simulink model "AttitudeKalman"  (Simulink 6.6)
settings: Solver=ode4  StartTime=0.0  StopTime=500  FixedStep=SampleT  RelTol=1e-3
InitFcn:
  | clc
  | Taxi_Var
  | failures
  | insInit
values from neighbouring files (symbols this model uses):
  A1 = 0    [Taxi_Var.m]    (also in Taxi_Var_new.m = 0.007)
  Apolar = 0.0899    [Taxi_Var.m]    (also in Taxi_Var_new.m = 0.057)
  APtsamp = 0.005    [failures.m]    (also in piccolo_init.m = 0.05)
  b0 = [0.01 0.01 0.01]    [insInit.m]
  CD0 = 0.0219    [Taxi_Var.m]    (also in Taxi_Var_new.m = 0.022)
  chord = S/span    (= 0.384036716878)    [Taxi_Var.m]    (also in Taxi_Var_new.m = 0.351341681574)
  CL0 = 0.1857    [Taxi_Var.m]    (also in Taxi_Var_new.m = 0.38)
  CLa = 4.6206    [Taxi_Var.m]    (also in Taxi_Var_new.m = 18.5)
  CLa_dot = 1.93    [Taxi_Var.m]    (also in Taxi_Var_new.m = 2.64)
  Clb = -0.0043    [Taxi_Var.m]    (also in Taxi_Var_new.m = -0.06)
  ClDa = 0.1695    [Taxi_Var.m]    (also in Taxi_Var_new.m)
  CLDe = 0.4032    [Taxi_Var.m]    (also in Taxi_Var_new.m = 0.24)
  CLDf = 0.047    [Taxi_Var.m]    (also in Taxi_Var_new.m = 0.4)
  ClDr = 0.0003    [Taxi_Var.m]    (also in Taxi_Var_new.m = 0.055)
  Clp = -0.4425    [Taxi_Var.m]    (also in Taxi_Var_new.m = -0.88)
  CLq = 8.7465    [Taxi_Var.m]    (also in Taxi_Var_new.m = 7.4)
  Clr = 0.0675    [Taxi_Var.m]    (also in Taxi_Var_new.m = 0.04)
  Cm0 = -0.0902    [Taxi_Var.m]    (also in Taxi_Var_new.m = 0.56)
  Cm0_factor = 0.9    [failures.m]
  Cm0_fail = 0    [failures.m]
  Cma = -1.3995    [Taxi_Var.m]    (also in Taxi_Var_new.m = -1.58)
  CmDe = -0.9493    [Taxi_Var.m]    (also in Taxi_Var_new.m = -41)
  CmDf = -.021    (= -0.021)    [Taxi_Var.m]    (also in Taxi_Var_new.m)
  Cnb = 0.0281    [Taxi_Var.m]    (also in Taxi_Var_new.m = 0.73)
  CnDa = -0.0031    [Taxi_Var.m]    (also in Taxi_Var_new.m = -0.032)
  CnDr = -0.0882    [Taxi_Var.m]    (also in Taxi_Var_new.m = 0.19)
  Cnp = -0.0695    [Taxi_Var.m]    (also in Taxi_Var_new.m = -0.1)
  Cnr = -0.1045    [Taxi_Var.m]    (also in Taxi_Var_new.m = -0.23)
  CYb = -0.1999    [Taxi_Var.m]    (also in Taxi_Var_new.m = -0.98)
  CYDr = 0.0192    [Taxi_Var.m]    (also in Taxi_Var_new.m = 0.066)
  da_failamp = 5    [failures.m]
  da_failbias = -da_failamp/2    (= -2.5)    [failures.m]
  da_failper = 90    [failures.m]
  daL_fail = 0    [failures.m]
  daR_fail = 0    [failures.m]
  dr_fail = 0    [failures.m]
  dr_failamp = 2    [failures.m]
  dr_failbias = -dr_failamp/2    (= -1)    [failures.m]
  dr_failper = 70    [failures.m]
  Euler_0 = [0; 0; 45]'*pi/180    [Taxi_Var.m]    (also in Taxi_Var_new.m = [0 0 45]'*pi/180)
  Gw = zeros(6,6)    [insInit.m]
  H = [eye(3,3) zeros(3,3)]    [insInit.m]
  ISA_g = 9.815    [Taxi_Var.m]    (also in Taxi_Var_new.m)
  Ixx = 3.689084    [Taxi_Var.m]    (also in Taxi_Var_new.m = 3.8)
  Iyy = 7.43789    [Taxi_Var.m]    (also in Taxi_Var_new.m = 9.58)
  Izz = 10.22202    [Taxi_Var.m]    (also in Taxi_Var_new.m = 9.68)
  mass = 22.5    [Taxi_Var.m]    (also in Taxi_Var_new.m = 8.16466266)
  MinThK = 0.075    [Taxi_Var.m]    (also in Taxi_Var_new.m = 0.077)
  P0 = diag([.3 .3 .3  .3 0.75 0.75 0.75 ])    [insInit.m]
  Pos_0 = [0; 0; 1000]'    [Taxi_Var.m]    (also in Taxi_Var_new.m = [0 0 500]')
  PQR_0 = [0; 0; 0]'    [Taxi_Var.m]    (also in Taxi_Var_new.m = [ 0 0 0]'*pi/180)
  Rv = rvv^2*eye(3)    [insInit.m]
  Rwpsd = zeros(6,6)    [insInit.m]
  SampleT = 0.005    [failures.m]
  span = 2.3368    [Taxi_Var.m]    (also in Taxi_Var_new.m = 2.795)
  tfailure = 20    [failures.m]
  ThK = 2.18    [Taxi_Var.m]    (also in Taxi_Var_new.m = 2.17)
  Vb_0 = [35; 0; 0]'    [Taxi_Var.m]    (also in Taxi_Var_new.m = [35 0 0]')
undefined symbols (not defined in the file or in its folder): clock, DiscIntNeverNeededParam, Earth, q0, sigbuilder_block, WGS84
libraries: simulink x25, aerolibconvert2 x6, aerolibactuator x6, dspsigops x5, aerolibutil x5, dspmtrx3 x4, aerolibtransform2 x2, aerolibatmos2 x2, aerolibnav x2, dspinverses x1
(part 1 of 2)
settings Model: Creator=ASL_Lab  LastModifiedBy=ASL_Lab
settings DebuggingCC: MultiTaskDSMMsg=warning  MultiTaskCondExecSysMsg=none  StrictBusMsg=None
settings HardwareCC: TargetHWDeviceType=32-bit Generic
settings RTWCC: IncludeERTFirstTime=on

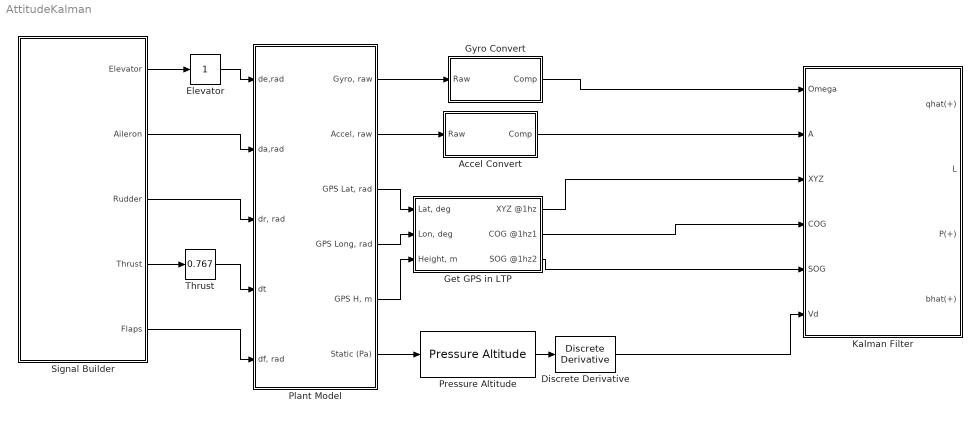
== system AttitudeKalman ==
  Accel Convert : Subsystem
  Discrete Derivative : simulink/Discrete/Discrete Derivative  SystemSampleTime=-1  gainval=1.0  ICPrevScaledInput=0.0  OutDataType=sfix(16)  OutScaling=2^-10  DoSatur=off
  Elevator : simulink/Math Operations/Slider Gain  SystemSampleTime=-1  low=-0.5  gain=1  high=1
  Get GPS in LTP : Subsystem
  Gyro Convert : Subsystem
  Kalman Filter : Subsystem
  Plant Model : Subsystem
  Pressure Altitude : aerolibatmos2/Pressure Altitude  SystemSampleTime=-1  units=Metric (MKS)  action=Warning
  Signal Builder : Subsystem  Tag=STV Subsys  LoadFcn=sigbuilder_block('load');  StartFcn=sigbuilder_block('start');  StopFcn=sigbuilder_block('stop');  ClipboardFcn=sigbuilder_block('clipboard');  mask(Sigbuilder block){}
      mask help: Sigbuilder GUI
      mask init:
      | if ~strcmp(get_param(bdroot(gcbh),'SimulationStatus'),'stopped') tuvar = sigbuilder_block('maskInit'); end
      settings: CopyFcn=sigbuilder_block('copy');  DeleteFcn=sigbuilder_block('delete');  ModelCloseFcn=sigbuilder_block('modelClose');  PreSaveFcn=sigbuilder_block('preSave');  NameChangeFcn=sigbuilder_block('namechange');  OpenFcn=sigbuilder_block('open',[3 3 762 514.5 ]);  CloseFcn=sigbuilder_block('close');
      mask Display: plot(0,0,100,100,[10,10,40,40,10],[80,20,20,80,80],[40,10],[50,50], [40,27,10],[65,72,56],[40,25,25,10],[28,28,43,43]);
  Thrust : simulink/Math Operations/Slider Gain  SystemSampleTime=-1  low=0  gain=0.767  high=1
  wires:
  Signal Builder/4(Thrust) -> Thrust/1
  Thrust/1 -> Plant Model/4(dt)
  Signal Builder/1(Elevator) -> Elevator/1
  Signal Builder/2(Aileron) -> Plant Model/2(da,rad)
  Signal Builder/3(Rudder) -> Plant Model/3("dr, rad")
  Signal Builder/5(Flaps) -> Plant Model/5("df, rad")
  Elevator/1 -> Plant Model/1(de,rad)
  Plant Model/1("Gyro, raw") -> Gyro Convert/1(Raw)
  Plant Model/2("Accel, raw") -> Accel Convert/1(Raw)
  Plant Model/3("GPS Lat, rad") -> Get GPS in LTP/1("Lat, deg")
  Plant Model/5("GPS H, m") -> Get GPS in LTP/3("Height, m")
  Plant Model/4("GPS Long, rad") -> Get GPS in LTP/2("Lon, deg")
  Gyro Convert/1(Comp) -> Kalman Filter/1(Omega)
  Get GPS in LTP/1(XYZ @1hz) -> Kalman Filter/3(XYZ)
  Accel Convert/1(Comp) -> Kalman Filter/2(A)
  Plant Model/6(Static (Pa)) -> Pressure Altitude/1
  Pressure Altitude/1 -> Discrete Derivative/1
  Discrete Derivative/1 -> Kalman Filter/6(Vd)
  Get GPS in LTP/2(COG @1hz1) -> Kalman Filter/4(COG)
  Get GPS in LTP/3(SOG @1hz2) -> Kalman Filter/5(SOG)

== system AttitudeKalman/Accel Convert ==
  Raw : Inport
  Bias : Constant  Value=[1866 1981 2042]
  Divide : Product  Inputs=/*  OutScaling=2^-10
  Gains : Constant  Value=[-142 142 235]
  Sum : Sum  Inputs=|+-
  Comp : Outport
  wires:
  Raw/1 -> Sum/1
  Divide/1 -> Comp/1
  Sum/1 -> Divide/2
  Gains/1 -> Divide/1
  Bias/1 -> Sum/2

== system AttitudeKalman/Get GPS in LTP ==
  "Lat, deg" : Inport
  "Lon, deg" : Inport  Port=2
  "Height, m" : Inport  Port=3
  Angle Conversion : aerolibconvert2/Angle Conversion  SystemSampleTime=-1  IU=rad  OU=deg
  Angle Conversion1 : aerolibconvert2/Angle Conversion  SystemSampleTime=-1  IU=rad  OU=deg
  Angle Conversion2 : aerolibconvert2/Angle Conversion  SystemSampleTime=-1  IU=rad  OU=deg
  Constant : Constant  Orientation=left  Value=[0 , 37.0004768371582, -122.061897277832]
  Demux : Demux  Outputs=3
  Demux1 : Demux  Outputs=3
  Discrete Derivative : simulink/Discrete/Discrete Derivative  SystemSampleTime=-1  gainval=1.0  ICPrevScaledInput=0.0  OutDataType=sfix(16)  OutScaling=2^-10  DoSatur=off
  Fcn : Fcn  Expr=sqrt(u(1)^2+u(2)^2+u(3)^2)
  Geod2LTP2 : Subsystem
      mask Description:
      | This block provides transformation of the Geodetic coordinates
      | to the LTP coorinate system. The block uses two consecutive transformations
      | (Geodetic -> ECEF ->LTP).
      | Geodetic coordinates of the LTP origin should also be predetermined.
      mask Help: Oops!
      mask Display: plot(0,0,100,100,[45,40,35,40,40],[85,95,85,95,40],[85,95,85,95,40],[35,40,45,40,40],[60,40,10,20,10,14],[70,40,10,13,10,20],[56,45],[70,70],[60,60],[50,60],[60,60],[30,40],[50,60],[20,20],[30,40],[20,20],[45,55],[35,25],[75,65],[35,25])
  Mux : Mux  Inputs=3
  Sim Latency : Subsystem
  Sim Latency3 : Subsystem
  Sim Latency4 : Subsystem
  Sim Latency5 : Subsystem
  Sim Latency6 : Subsystem
  Trigonometric Function : Trigonometry  Operator=atan2
  XYZ @1hz : Outport
  COG @1hz1 : Outport  Port=2
  SOG @1hz2 : Outport  Port=3
  wires:
  Constant/1 -> Geod2LTP2/1("Height, Lat, Lon Initials from GPS")
  Geod2LTP2/1("NEU, m") -> Discrete Derivative/1, Demux1/1
  "Lat, deg"/1 -> Angle Conversion1/1
  "Lon, deg"/1 -> Angle Conversion2/1
  "Height, m"/1 -> Geod2LTP2/4(Hight,m(GPS))
  Fcn/1 -> Sim Latency6/1(Fast Data)
  Demux/2 -> Trigonometric Function/1
  Demux/1 -> Trigonometric Function/2
  Trigonometric Function/1 -> Angle Conversion/1
  Angle Conversion/1 -> Sim Latency5/1(Fast Data)
  Discrete Derivative/1 -> Demux/1, Fcn/1
  Mux/1 -> XYZ @1hz/1
  Angle Conversion1/1 -> Geod2LTP2/2("Lat, deg(GPS)")
  Angle Conversion2/1 -> Geod2LTP2/3("Lon, deg(GPS)")
  Demux1/1 -> Sim Latency/1(Fast Data)
  Demux1/2 -> Sim Latency3/1(Fast Data)
  Demux1/3 -> Sim Latency4/1(Fast Data)
  Sim Latency/1(1Hz Data) -> Mux/1
  Sim Latency3/1(1Hz Data) -> Mux/2
  Sim Latency4/1(1Hz Data) -> Mux/3
  Sim Latency5/1(1Hz Data) -> COG @1hz1/1
  Sim Latency6/1(1Hz Data) -> SOG @1hz2/1

== system AttitudeKalman/Gyro Convert ==
  Raw : Inport
  Bias : Constant  Value=[1866 1981 2042]
  Divide : Product  Inputs=/*  OutScaling=2^-10
  Gains : Constant  Value=[-142 142 235]
  Sum : Sum  Inputs=|+-
  Comp : Outport
  wires:
  Bias/1 -> Sum/2
  Gains/1 -> Divide/1
  Sum/1 -> Divide/2
  Divide/1 -> Comp/1
  Raw/1 -> Sum/1

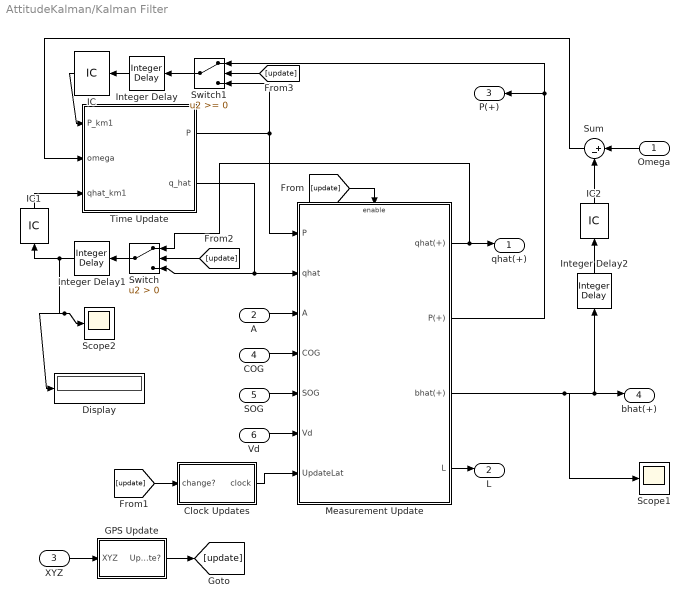
== system AttitudeKalman/Kalman Filter ==
  Omega : Inport  Orientation=left
  A : Inport  Port=2
  XYZ : Inport  Port=3
  COG : Inport  Port=4
  SOG : Inport  Port=5
  Vd : Inport  Port=6
  Clock Updates : Subsystem
  Display : Display
  GPS Update : Subsystem
  IC : InitialCondition  Orientation=left  Value=P0
  IC1 : InitialCondition  Orientation=up  Value=q0
  IC2 : InitialCondition  Orientation=up  Value=b0
  Integer Delay : simulink/Discrete/Integer Delay  Orientation=left  vinit=0.0  samptime=SampleT  NumDelays=1
  Integer Delay1 : simulink/Discrete/Integer Delay  Orientation=left  vinit=0.0  samptime=SampleT  NumDelays=1
  Integer Delay2 : simulink/Discrete/Integer Delay  Orientation=up  vinit=0.0  samptime=SampleT  NumDelays=1
  Measurement Update : Subsystem
  Scope1 : Scope
      settings: SaveName=ScopeData3
  Scope2 : Scope
      settings: YMin=-0.9  YMax=0.4  SaveName=ScopeData4
  Sum : Sum  Orientation=left  Inputs=|+-
  Switch : Switch  Orientation=left  Criteria=u2 > Threshold
  Switch1 : Switch  Orientation=left
  Time Update : Subsystem
  qhat(+) : Outport
  L : Outport  Port=2
  P(+) : Outport  Orientation=left  Port=3
  bhat(+) : Outport  Port=4
  wires:
  Integer Delay/1 -> IC/1
  Time Update/1(P) -> Measurement Update/1(P), Switch1/3
  Time Update/2(q_hat) -> Measurement Update/2(qhat), Switch/3
  XYZ/1 -> GPS Update/1(XYZ)
  A/1 -> Measurement Update/3(A)
  COG/1 -> Measurement Update/4(COG)
  SOG/1 -> Measurement Update/5(SOG)
  Vd/1 -> Measurement Update/6(Vd)
  GPS Update/1(Update?) -> [update]
  [update] -> Measurement Update/Enable
  Clock Updates/1(clock) -> Measurement Update/7(UpdateLat)
  [update] -> Clock Updates/1(change?)
  Measurement Update/1(qhat(+)) -> qhat(+)/1, Switch/1
  [update] -> Switch/2
  Switch/1 -> Integer Delay1/1
  Integer Delay1/1 -> IC1/1, Scope2/1, Display/1
  [update] -> Switch1/2
  Switch1/1 -> Integer Delay/1
  Measurement Update/2(P(+)) -> Switch1/1, P(+)/1
  Omega/1 -> Sum/1
  Measurement Update/3(bhat(+)) -> bhat(+)/1, Integer Delay2/1, Scope1/1
  Sum/1 -> Time Update/2(omega)
  Measurement Update/4(L) -> L/1
  Integer Delay2/1 -> IC2/1
  IC/1 -> Time Update/1(P_km1)
  IC1/1 -> Time Update/3(qhat_km1)
  IC2/1 -> Sum/2

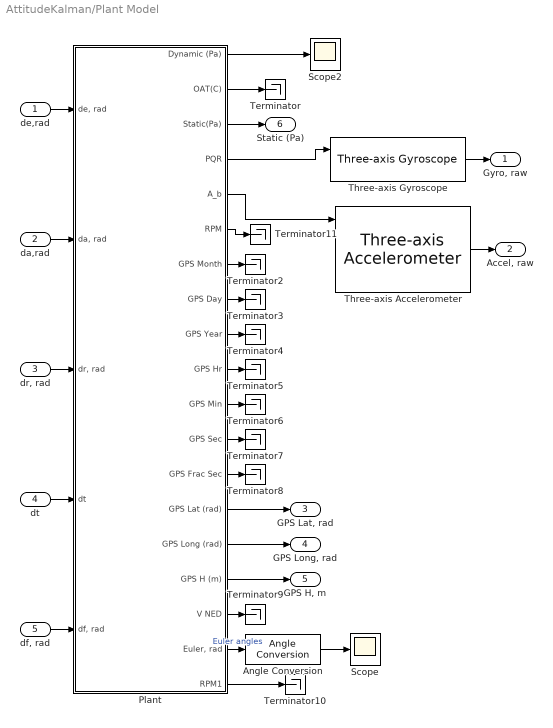
== system AttitudeKalman/Plant Model ==
  de,rad : Inport
  da,rad : Inport  Port=2
  "dr, rad" : Inport  Port=3
  dt : Inport  Port=4
  "df, rad" : Inport  Port=5
  Angle Conversion : aerolibconvert2/Angle Conversion  SystemSampleTime=-1  IU=rad  OU=deg
  Plant : Subsystem
  Scope : Scope
      settings: TimeRange=300  YMin=-0.8  YMax=0.6000000000000001
  Scope2 : Scope
      settings: TimeRange=300  YMin=350  YMax=625  SaveName=ScopeData16
  Terminator{,2..11} (11 alike) : Terminator
  Three-axis Accelerometer : aerolibnav/Three-axis Accelerometer  SystemSampleTime=-1  units=Metric (MKS)  acc=[0 0 0]  gtype=off  dtype_a=on  w_a=190  z_a=0.707  a_sf_cc=[-41 0 0; 0 41 0; 0 0 -43]  a_bias=[2015 2018 2006]  a_rand=on  a_seeds=[23093 23094 23095]  a_pow=[0.008 0.008 0.008]  a_sat="[-inf  -inf  -inf  inf inf inf]"  a_Ts=SampleT
  Three-axis Gyroscope : aerolibnav/Three-axis Gyroscope  SystemSampleTime=-1  dtype_g=on  w_g=190  z_g=0.707  g_sf_cc=[-147 0 0; 0 132 0; 0 0 205]  g_bias=[1866 1981 2042]  g_sen=[0 0 0]  g_rand=on  g_seeds=[23093 23094 23095]  g_pow=[0.008 0.008 0.008]  g_sat="[-inf  -inf  -inf  inf inf inf]"  g_Ts=SampleT
  "Gyro, raw" : Outport
  "Accel, raw" : Outport  Port=2
  "GPS Lat, rad" : Outport  Port=3
  "GPS Long, rad" : Outport  Port=4
  "GPS H, m" : Outport  Port=5
  Static (Pa) : Outport  Port=6
  wires:
  Plant/17(V NED) -> Terminator9/1
  Plant/13(GPS Frac Sec) -> Terminator8/1
  Plant/12(GPS Sec) -> Terminator7/1
  Plant/11(GPS Min) -> Terminator6/1
  Plant/10(GPS Hr) -> Terminator5/1
  Plant/9(GPS Year) -> Terminator4/1
  Plant/8(GPS Day) -> Terminator3/1
  Plant/7(GPS Month) -> Terminator2/1
  Plant/3(Static(Pa)) -> Static (Pa)/1
  Plant/2(OAT(C)) -> Terminator/1
  Plant/5(A_b) -> Three-axis Accelerometer/1
  Plant/4(PQR) -> Three-axis Gyroscope/1
  Plant/1(Dynamic (Pa)) -> Scope2/1
  Plant/18("Euler, rad") -> Angle Conversion/1  "Euler angles"
  de,rad/1 -> Plant/1("de, rad")
  Three-axis Gyroscope/1 -> "Gyro, raw"/1
  Plant/6(RPM) -> Terminator11/1
  da,rad/1 -> Plant/2("da, rad")
  Three-axis Accelerometer/1 -> "Accel, raw"/1
  "dr, rad"/1 -> Plant/3("dr, rad")
  dt/1 -> Plant/4(dt)
  "df, rad"/1 -> Plant/5("df, rad")
  Plant/19(RPM1) -> Terminator10/1
  Angle Conversion/1 -> Scope/1
  Plant/14(GPS Lat (rad)) -> "GPS Lat, rad"/1
  Plant/15(GPS Long (rad)) -> "GPS Long, rad"/1
  Plant/16(GPS H (m)) -> "GPS H, m"/1

== system AttitudeKalman/Signal Builder ==
  Demux : Demux  Tag=STV Demux  Outputs=5
  FromWs : FromWorkspace  Tag=STV FromWs  VariableName=tuvar  SampleTime=0  SigBuilderData=DataTag0  VnvData=DataTag1
      SigBuilderData=|
      | channels(1).label = 'Elevator'
      | channels(1).allXData = {[0 200], [0 200], [0 100 100 200]}
      | channels(1).allYData = {[0.2 0.2], [-0.07 -0.07], [-0.07 -0.07 0 -0.07]}
      | channels(2).label = 'Aileron'
      | channels(2).allXData = {[0 80 80.01 84 84.01 88 88.01 200], [0 200], [0 200]}
      | channels(2).allYData = {[0 0 3 3 -3 -3 0 0], [0 0], [0 0]}
      | channels(3).label = 'Rudder'
      | channels(3).allXData = {[0 200], [0 200], [0 200]}
      | channels(3).allYData = {[0 0], [0 0], [0 0]}
      | channels(4).label = 'Thrust'
      | channels(4).allXData = {[0 200], [0 200], [0 200]}
      | channels(4).allYData = {[0.125 0.125], [1 1], [1 1]}
      | channels(5).label = 'Flaps'
      | channels(5).allXData = {[0 200], [0 200], [0 200]}
      | channels(5).allYData = {[0 0], [0 0], [0 0]}
      | common.afterFinalStr = 'Extrapolate'
      | common.sampleTime = 0
      | dataSet(1).timeRange = [0 200]
      | dataSet(1).name = 'Aileron 5 Deg'
      | dataSet(2).timeRange = [0 200]
      | dataSet(2).name = 'Trim'
      | dataSet(3).timeRange = [0 200]
      | dataSet(3).name = 'Elevator'
  Elevator : Outport  Tag=STV Outport
  Aileron : Outport  Tag=STV Outport  Port=2
  Rudder : Outport  Tag=STV Outport  Port=3
  Thrust : Outport  Tag=STV Outport  Port=4
  Flaps : Outport  Tag=STV Outport  Port=5
  wires:
  Demux/1 -> Elevator/1
  FromWs/1 -> Demux/1
  Demux/2 -> Aileron/1
  Demux/3 -> Rudder/1
  Demux/4 -> Thrust/1
  Demux/5 -> Flaps/1

== system AttitudeKalman/Get GPS in LTP/Geod2LTP2 ==
  "Height, Lat, Lon Initials from GPS" : Inport
  "Lat, deg(GPS)" : Inport  Port=2
  "Lon, deg(GPS)" : Inport  Port=3
  Hight,m(GPS) : Inport  Port=4
  Demux : Demux  Outputs=3
  ECEF2LTP (UEN) : Subsystem
      mask Display: plot(0,0,100,100,[45,40,35,40,40],[85,95,85,95,40],[85,95,85,95,40],[35,40,45,40,40],[60,40,10,20,10,14],[70,40,10,13,10,20],[56,45],[70,70],[60,60],[50,60],[60,60],[30,40],[50,60],[20,20],[30,40],[20,20],[45,55],[35,25],[75,65],[35,25])
  Geod2ECEF : Subsystem  mask{Re=6378137, Rp=6356752.3142}
      mask prompts: Re "Enter equatorial radius, m"; Rp "Enter polar radius,m"
  Geod2ECEF1 : Subsystem  mask{Re=6378137, Rp=6356752.3142}
      mask prompts: Re "Enter equatorial radius, m"; Rp "Enter polar radius,m"
  Mux : Mux  Inputs=3
  Mux1 : Mux  Inputs=2
  Mux2 : Mux  Inputs=3
  Reshape : Reshape  OutputDimensionality=Column vector (2-D)
  Sum1 : Sum  Inputs=|+-  SaturateOnIntegerOverflow=on
  UEN 2 NEU : Gain  Gain=[0 0 1;0 1 0;1 0 0]  Multiplication=Matrix(K*u)  SaturateOnIntegerOverflow=on
  "NEU, m" : Outport
  wires:
  UEN 2 NEU/1 -> "NEU, m"/1
  Geod2ECEF/3("Ze, m ") -> Mux/3
  Geod2ECEF/1("Xe, m ") -> Mux/1
  Geod2ECEF/2("Ye, m ") -> Mux/2
  "Lat, deg(GPS)"/1 -> Geod2ECEF/2("lat, deg")
  "Lon, deg(GPS)"/1 -> Geod2ECEF/3(lon,deg)
  Mux1/1 -> ECEF2LTP (UEN)/2("Long, Lat")
  Geod2ECEF1/3("Ze, m ") -> Mux2/3
  Geod2ECEF1/1("Xe, m ") -> Mux2/1
  Geod2ECEF1/2("Ye, m ") -> Mux2/2
  Mux2/1 -> Sum1/2  "R_in"
  Demux/1 -> Geod2ECEF1/1("height, m")
  Demux/2 -> Mux1/2, Geod2ECEF1/2("lat, deg")
  Demux/3 -> Mux1/1, Geod2ECEF1/3(lon,deg)
  ECEF2LTP (UEN)/1(Out) -> Reshape/1  "Moving Side"
  Hight,m(GPS)/1 -> Geod2ECEF/1("height, m")
  "Height, Lat, Lon Initials from GPS"/1 -> Demux/1
  Mux/1 -> Sum1/1  "r_mov"
  Sum1/1 -> ECEF2LTP (UEN)/1(ECEF coordinates)
  Reshape/1 -> UEN 2 NEU/1

== system AttitudeKalman/Get GPS in LTP/Sim Latency ==
  Fast Data : Inport
  Counter Free-Running1 : simulink/Sources/Counter Free-Running  SystemSampleTime=-1  NumBits=1  tsamp=1
  Rate Transition2 : RateTransition  OutPortSampleTime=SampleT
  Sample and Hold : dspsigops/Sample and Hold  SystemSampleTime=-1  trig=Either edge  initCond=0  latchinput=off
  1Hz Data : Outport
  wires:
  Sample and Hold/1 -> 1Hz Data/1
  Fast Data/1 -> Sample and Hold/1
  Rate Transition2/1 -> Sample and Hold/Trigger
  Counter Free-Running1/1 -> Rate Transition2/1

== system AttitudeKalman/Get GPS in LTP/Sim Latency3 ==
  Fast Data : Inport
  Counter Free-Running1 : simulink/Sources/Counter Free-Running  SystemSampleTime=-1  NumBits=1  tsamp=1
  Rate Transition2 : RateTransition  OutPortSampleTime=SampleT
  Sample and Hold : dspsigops/Sample and Hold  SystemSampleTime=-1  trig=Either edge  initCond=0  latchinput=off
  1Hz Data : Outport
  wires:
  Counter Free-Running1/1 -> Rate Transition2/1
  Rate Transition2/1 -> Sample and Hold/Trigger
  Fast Data/1 -> Sample and Hold/1
  Sample and Hold/1 -> 1Hz Data/1

== system AttitudeKalman/Get GPS in LTP/Sim Latency4 ==
  Fast Data : Inport
  Counter Free-Running1 : simulink/Sources/Counter Free-Running  SystemSampleTime=-1  NumBits=1  tsamp=1
  Rate Transition2 : RateTransition  OutPortSampleTime=SampleT
  Sample and Hold : dspsigops/Sample and Hold  SystemSampleTime=-1  trig=Either edge  initCond=0  latchinput=off
  1Hz Data : Outport
  wires:
  Sample and Hold/1 -> 1Hz Data/1
  Fast Data/1 -> Sample and Hold/1
  Rate Transition2/1 -> Sample and Hold/Trigger
  Counter Free-Running1/1 -> Rate Transition2/1

== system AttitudeKalman/Get GPS in LTP/Sim Latency5 ==
  Fast Data : Inport
  Counter Free-Running1 : simulink/Sources/Counter Free-Running  SystemSampleTime=-1  NumBits=1  tsamp=1
  Rate Transition2 : RateTransition  OutPortSampleTime=SampleT
  Sample and Hold : dspsigops/Sample and Hold  SystemSampleTime=-1  trig=Either edge  initCond=0  latchinput=off
  1Hz Data : Outport
  wires:
  Counter Free-Running1/1 -> Rate Transition2/1
  Rate Transition2/1 -> Sample and Hold/Trigger
  Fast Data/1 -> Sample and Hold/1
  Sample and Hold/1 -> 1Hz Data/1

== system AttitudeKalman/Get GPS in LTP/Sim Latency6 ==
  Fast Data : Inport
  Counter Free-Running1 : simulink/Sources/Counter Free-Running  SystemSampleTime=-1  NumBits=1  tsamp=1
  Rate Transition2 : RateTransition  OutPortSampleTime=SampleT
  Sample and Hold : dspsigops/Sample and Hold  SystemSampleTime=-1  trig=Either edge  initCond=0  latchinput=off
  1Hz Data : Outport
  wires:
  Sample and Hold/1 -> 1Hz Data/1
  Fast Data/1 -> Sample and Hold/1
  Rate Transition2/1 -> Sample and Hold/Trigger
  Counter Free-Running1/1 -> Rate Transition2/1

== system AttitudeKalman/Kalman Filter/Clock Updates ==
  change? : Inport
  Constant : Constant
  Constant1 : Constant  Value=0
  Constant2 : Constant  Value=SampleT
  Discrete-Time Integrator : DiscreteIntegrator  ExternalReset=rising  InitialConditionSource=external  SampleTime=SampleT  ICPrevOutput=DiscIntNeverNeededParam  ICPrevScaledInput=DiscIntNeverNeededParam
  Integer Delay2 : simulink/Discrete/Integer Delay  vinit=0.0  samptime=-1  NumDelays=1
  Sum : Sum  Inputs=|++
  clock : Outport
  wires:
  Sum/1 -> clock/1
  Constant2/1 -> Sum/2
  Integer Delay2/1 -> Sum/1
  change?/1 -> Discrete-Time Integrator/2
  Discrete-Time Integrator/1 -> Integer Delay2/1
  Constant1/1 -> Discrete-Time Integrator/3
  Constant/1 -> Discrete-Time Integrator/1

== system AttitudeKalman/Kalman Filter/GPS Update ==
  XYZ : Inport
  Demux : Demux  Outputs=3
  Detect Change : Subsystem
  Detect Change1 : Subsystem
  Detect Change2 : Subsystem
  Saturation1 : Saturate  UpperLimit=1  LowerLimit=0  SampleTime=SampleT
  Sum : Sum  Inputs=3
  Update? : Outport
  wires:
  Demux/1 -> Detect Change/1(Data)
  Demux/2 -> Detect Change1/1(Data)
  Demux/3 -> Detect Change2/1(Data)
  Detect Change/1(change?) -> Sum/1
  Detect Change1/1(change?) -> Sum/2
  Detect Change2/1(change?) -> Sum/3
  Sum/1 -> Saturation1/1
  XYZ/1 -> Demux/1
  Saturation1/1 -> Update?/1

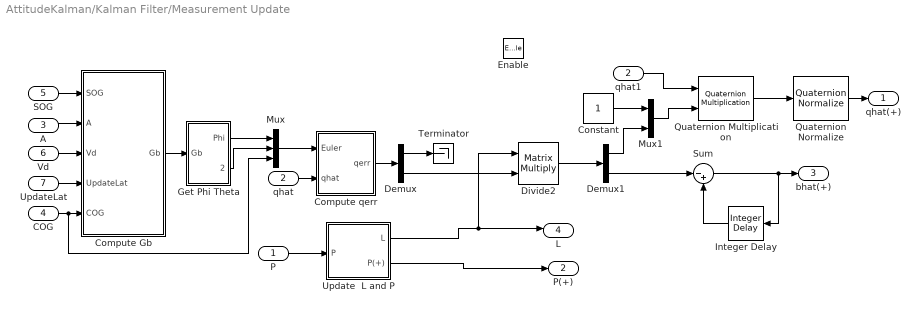
== system AttitudeKalman/Kalman Filter/Measurement Update ==
  P : Inport
  qhat : Inport  Port=2
  A : Inport  Port=3
  COG : Inport  Port=4
  SOG : Inport  Port=5
  Vd : Inport  Port=6
  UpdateLat : Inport  Port=7
  Enable : EnablePort
  Compute Gb : Subsystem
  Compute qerr : Subsystem
  Constant : Constant
  Demux : Demux  Outputs=[1 3]
  Demux1 : Demux  Outputs=[3 3]
  Divide2 : Product  Multiplication=Matrix(*)  OutScaling=2^-10
  Get Phi Theta : Subsystem
  Integer Delay : simulink/Discrete/Integer Delay  Orientation=left  vinit=0.0  samptime=-1  NumDelays=1
  Mux : Mux  Inputs=3
  Mux1 : Mux  Inputs=2
  Quaternion Multiplication : aerolibutil/Quaternion Multiplication  SystemSampleTime=-1
  Quaternion Normalize : aerolibutil/Quaternion Normalize  SystemSampleTime=-1
  Sum : Sum  Inputs=|-+
  Terminator : Terminator
  Update  L and P : Subsystem
  qhat1 : InportShadow  Port=2  LatchByCopyingInsideSignal=off
  qhat(+) : Outport
  P(+) : Outport  Port=2
  bhat(+) : Outport  Port=3
  L : Outport  Port=4
  wires:
  SOG/1 -> Compute Gb/1(SOG)
  A/1 -> Compute Gb/2(A)
  Vd/1 -> Compute Gb/3(Vd)
  UpdateLat/1 -> Compute Gb/4(UpdateLat)
  COG/1 -> Compute Gb/5(COG), Mux/3
  Compute Gb/1(Gb) -> Get Phi Theta/1(Gb)
  Get Phi Theta/1(Phi) -> Mux/1
  Get Phi Theta/2(Theta) -> Mux/2
  Mux/1 -> Compute qerr/1(Euler)
  qhat/1 -> Compute qerr/2(qhat)
  P/1 -> Update  L and P/1(P)
  Update  L and P/1(L) -> L/1, Divide2/1
  Update  L and P/2(P(+)) -> P(+)/1
  Compute qerr/1(qerr) -> Demux/1
  Divide2/1 -> Demux1/1
  Demux1/1 -> Mux1/2
  Constant/1 -> Mux1/1
  Mux1/1 -> Quaternion Multiplication/2
  qhat1/1 -> Quaternion Multiplication/1
  Quaternion Multiplication/1 -> Quaternion Normalize/1
  Quaternion Normalize/1 -> qhat(+)/1
  Demux1/2 -> Sum/1
  Sum/1 -> bhat(+)/1, Integer Delay/1
  Integer Delay/1 -> Sum/2
  Demux/2 -> Divide2/2
  Demux/1 -> Terminator/1

== system AttitudeKalman/Kalman Filter/Time Update ==
  P_km1 : Inport
  omega : Inport  Port=2
  qhat_km1 : Inport  Port=3
  Constant1 : Constant  Value=SampleT
  Discrete-Time Integrator : DiscreteIntegrator  InitialCondition=q0  SampleTime=SampleT  ICPrevOutput=DiscIntNeverNeededParam  ICPrevScaledInput=DiscIntNeverNeededParam
  Divide : Product  OutScaling=2^-10
  Divide1 : Product  Inputs=3  Multiplication=Matrix(*)  OutScaling=2^-10
  Divide2 : Product  Multiplication=Matrix(*)  OutScaling=2^-10
  Embedded MATLAB Function : Stateflow chart
  Embedded MATLAB Function1 : Stateflow chart
  Gain : Gain  Gain=0.5
  Matrix Exponential : dspmtrx3/Matrix Exponential  SystemSampleTime=-1
  Quaternion Normalize : aerolibutil/Quaternion Normalize  SystemSampleTime=-1
  Subsystem : Subsystem
  Sum : Sum  Inputs=|++
  Transpose : dspmtrx3/Transpose  SystemSampleTime=-1  Hermitian=off  overflowFlag=off
  P : Outport
  q_hat : Outport  Port=2
  wires:
  Embedded MATLAB Function/1(F) -> Divide/1
  Constant1/1 -> Divide/2
  Divide/1 -> Matrix Exponential/1
  omega/1 -> Embedded MATLAB Function1/1(omega), Embedded MATLAB Function/1(omega)
  Matrix Exponential/1 -> Divide1/1, Transpose/1
  Transpose/1 -> Divide1/3
  Divide1/1 -> Sum/1
  Subsystem/1(Cd) -> Sum/2
  Embedded MATLAB Function1/1(O) -> Gain/1
  Divide2/1 -> Discrete-Time Integrator/1
  Gain/1 -> Divide2/1
  P_km1/1 -> Divide1/2
  Sum/1 -> P/1
  Discrete-Time Integrator/1 -> Quaternion Normalize/1
  qhat_km1/1 -> Divide2/2
  Quaternion Normalize/1 -> q_hat/1

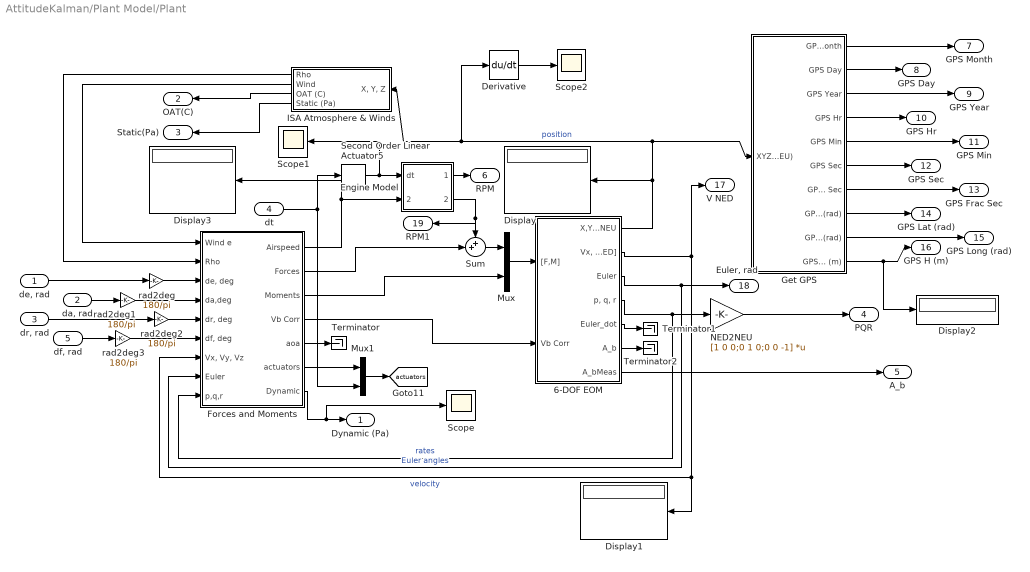
== system AttitudeKalman/Plant Model/Plant ==
  "de, rad" : Inport  OutDataType=fixdt(1,16,0)  OutScaling=[]
  "da, rad" : Inport  Port=2  OutDataType=fixdt(1,16,0)  OutScaling=[]
  "dr, rad" : Inport  Port=3  OutDataType=fixdt(1,16,0)  OutScaling=[]
  dt : Inport  Port=4  OutDataType=fixdt(1,16,0)  OutScaling=[]
  "df, rad" : Inport  Port=5  OutDataType=fixdt(1,16,0)  OutScaling=[]
  6-DOF EOM : Subsystem
  Derivative : Derivative
  Display{,1..3} (4 alike) : Display
  Engine Model : Subsystem
  Forces and Moments : Subsystem
  Get GPS : Subsystem
  ISA Atmosphere & Winds : Subsystem  Orientation=left
  Mux : Mux  Inputs=2
  Mux1 : Mux  Inputs=2
  "NED2NEU " : Gain  Gain=[1 0 0;0 1 0;0 0 -1]  Multiplication=Matrix(K*u)  SaturateOnIntegerOverflow=on
  Scope : Scope
      settings: YMin=350  YMax=650  SaveName=ScopeData2
  Scope1 : Scope
      settings: YMin=0.999987  YMax=0.999987  SaveName=ScopeData14
  Scope2 : Scope
      settings: YMin=350  YMax=650  SaveName=ScopeData23
  Second Order Linear Actuator5 : aerolibactuator/Second Order Linear Actuator  SystemSampleTime=-1  wn_fin=10  z_fin=0.7  fin_act_0=0
  Sum : Sum  Inputs=++|  SaturateOnIntegerOverflow=on
  Terminator : Terminator
  Terminator1 : Terminator
  Terminator2 : Terminator
  rad2deg{,1..3} (4 alike) : Gain  Gain=180/pi  SaturateOnIntegerOverflow=on
  Dynamic (Pa) : Outport
  OAT(C) : Outport  Orientation=left  Port=2
  Static(Pa) : Outport  Orientation=left  Port=3
  PQR : Outport  Port=4
  A_b : Outport  Port=5
  RPM : Outport  Port=6
  GPS Month : Outport  Port=7
  GPS Day : Outport  Port=8
  GPS Year : Outport  Port=9
  GPS Hr : Outport  Port=10
  GPS Min : Outport  Port=11
  GPS Sec : Outport  Port=12
  GPS Frac Sec : Outport  Port=13
  GPS Lat (rad) : Outport  Port=14
  GPS Long (rad) : Outport  Port=15
  GPS H (m) : Outport  Port=16
  V NED : Outport  Port=17
  "Euler, rad" : Outport  Port=18
  RPM1 : Outport  Orientation=left  Port=19
  tag scope: actuators=global
  wires:
  6-DOF EOM/4("p, q, r") -> Forces and Moments/9(p,q,r), "NED2NEU "/1  "rates"
  6-DOF EOM/3(Euler) -> "Euler, rad"/1, Forces and Moments/8(Euler)  "Euler angles"
  6-DOF EOM/2("Vx, Vy, Vz [NED]") -> V NED/1, Forces and Moments/7("Vx, Vy, Vz "), Display1/1  "velocity"
  Engine Model/1(RPM) -> RPM/1
  6-DOF EOM/1(X,Y,Z (LTP) NEU) -> Get GPS/1(XYZ (NEU)), ISA Atmosphere & Winds/1("X, Y, Z"), Derivative/1, Display/1  "position"
  Forces and Moments/4(Vb Corr) -> 6-DOF EOM/2(Vb Corr)
  Mux/1 -> 6-DOF EOM/1("[F,M]")
  Sum/1 -> Mux/1
  Forces and Moments/2(Forces) -> Sum/2
  Forces and Moments/3(Moments) -> Mux/2
  ISA Atmosphere & Winds/1(Rho) -> Forces and Moments/2(Rho)
  ISA Atmosphere & Winds/2(Wind) -> Forces and Moments/1(Wind e)
  Forces and Moments/5(aoa) -> Terminator/1
  rad2deg/1 -> Forces and Moments/3("de, deg")
  rad2deg1/1 -> Forces and Moments/4(da,deg)
  rad2deg2/1 -> Forces and Moments/5("dr, deg")
  rad2deg3/1 -> Forces and Moments/6("df, deg")
  Forces and Moments/6(actuators) -> Mux1/1
  Mux1/1 -> [actuators]
  dt/1 -> Mux1/2, Second Order Linear Actuator5/1
  "de, rad"/1 -> rad2deg/1
  "da, rad"/1 -> rad2deg1/1
  "dr, rad"/1 -> rad2deg2/1
  "df, rad"/1 -> rad2deg3/1
  Forces and Moments/7(Dynamic) -> Dynamic (Pa)/1, Scope/1
  ISA Atmosphere & Winds/3(OAT (C)) -> OAT(C)/1
  ISA Atmosphere & Winds/4(Static (Pa)) -> Static(Pa)/1
  Engine Model/2(Thrust) -> Sum/1, RPM1/1
  Get GPS/1(GPS Month) -> GPS Month/1
  Get GPS/2(GPS Day) -> GPS Day/1
  Get GPS/3(GPS Year) -> GPS Year/1
  Get GPS/4(GPS Hr) -> GPS Hr/1
  Get GPS/5(GPS Min) -> GPS Min/1
  Get GPS/6(GPS Sec) -> GPS Sec/1
  Get GPS/7(GPS Frac Sec) -> GPS Frac Sec/1
  Get GPS/8(GPS Lat (rad)) -> GPS Lat (rad)/1
  Get GPS/9(GPS Long (rad)) -> GPS Long (rad)/1
  Get GPS/10(GPS H (m)) -> GPS H (m)/1, Display2/1
  6-DOF EOM/5(Euler_dot) -> Terminator1/1
  "NED2NEU "/1 -> PQR/1
  Forces and Moments/1(Airspeed) -> Engine Model/2(Vmag), Display3/1
  Second Order Linear Actuator5/1 -> Engine Model/1(dt), Scope1/1
  6-DOF EOM/7(A_bMeas) -> A_b/1
  Derivative/1 -> Scope2/1
  6-DOF EOM/6(A_b) -> Terminator2/1

== system AttitudeKalman/Get GPS in LTP/Geod2LTP2/ECEF2LTP (UEN) ==
  ECEF coordinates : Inport
  "Long, Lat" : Inport  Port=2
  Deg2R : Gain  Gain=pi/180  SaturateOnIntegerOverflow=on
  Demux3 : Demux  Outputs=2
  From Body to Universal1 : Subsystem
  Product1 : Product  Multiplication=Matrix(*)  SaturateOnIntegerOverflow=on  InputSameDT=on
  Out : Outport
  wires:
  "Long, Lat"/1 -> Deg2R/1
  Product1/1 -> Out/1
  Demux3/2 -> From Body to Universal1/2(lat)
  Demux3/1 -> From Body to Universal1/1(long)
  Deg2R/1 -> Demux3/1
  ECEF coordinates/1 -> Product1/2
  From Body to Universal1/1(DCM) -> Product1/1

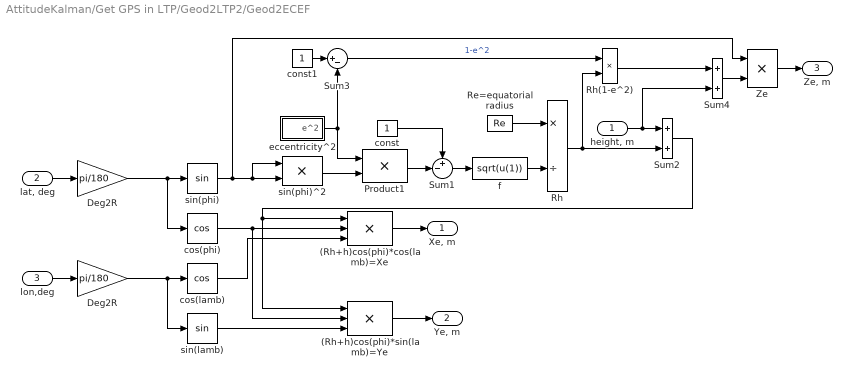
== system AttitudeKalman/Get GPS in LTP/Geod2LTP2/Geod2ECEF ==
  "height, m" : Inport
  "lat, deg" : Inport  Port=2
  lon,deg : Inport  Port=3
  (Rh+h)cos(phi)*cos(lamb)=Xe : Product  Inputs=3  SaturateOnIntegerOverflow=on  InputSameDT=on
  (Rh+h)cos(phi)*sin(lamb)=Ye : Product  Inputs=3  SaturateOnIntegerOverflow=on  InputSameDT=on
  Deg2R : Gain  Gain=pi/180  SaturateOnIntegerOverflow=on
  "Deg2R " : Gain  Gain=pi/180  SaturateOnIntegerOverflow=on
  Product1 : Product  SaturateOnIntegerOverflow=on  InputSameDT=on
  Re=equatorial radius : Constant  Value=Re
  Rh : Product  Inputs=*/  SaturateOnIntegerOverflow=on  InputSameDT=on
  Rh(1-e^2) : Product  SaturateOnIntegerOverflow=on  InputSameDT=on
  Sum1 : Sum  Inputs=+-|  SaturateOnIntegerOverflow=on  InputSameDT=on
  Sum2 : Sum  SaturateOnIntegerOverflow=on  InputSameDT=on
      settings: AttributesFormatString=Rh+h
  Sum3 : Sum  Inputs=|+-  SaturateOnIntegerOverflow=on  InputSameDT=on
  Sum4 : Sum  SaturateOnIntegerOverflow=on  InputSameDT=on
      settings: AttributesFormatString=(1-e^2)Rh+h
  Ze : Product  SaturateOnIntegerOverflow=on  InputSameDT=on
  const : Constant
  const1 : Constant
  cos(lamb) : Trigonometry  Operator=cos
  cos(phi) : Trigonometry  Operator=cos
  eccentricity^2 : Subsystem
  f : Fcn  Expr=sqrt(u(1))
  sin(lamb) : Trigonometry
  sin(phi) : Trigonometry
  sin(phi)^2 : Product  SaturateOnIntegerOverflow=on  InputSameDT=on
  "Xe, m " : Outport
  "Ye, m " : Outport  Port=2
  "Ze, m " : Outport  Port=3
  wires:
  "lat, deg"/1 -> Deg2R/1
  sin(phi)/1 -> sin(phi)^2/1, sin(phi)^2/2, Ze/1
  f/1 -> Rh/2
  Re=equatorial radius/1 -> Rh/1
  Rh/1 -> Sum2/2, Rh(1-e^2)/2
  Product1/1 -> Sum1/2
  Sum1/1 -> f/1
  const/1 -> Sum1/1
  "height, m"/1 -> Sum4/2, Sum2/1
  eccentricity^2/1(e^2) -> Product1/1, Sum3/2
  sin(phi)^2/1 -> Product1/2
  const1/1 -> Sum3/1
  Sum3/1 -> Rh(1-e^2)/1  "1-e^2"
  Rh(1-e^2)/1 -> Sum4/1
  Sum4/1 -> Ze/2
  lon,deg/1 -> "Deg2R "/1
  cos(phi)/1 -> (Rh+h)cos(phi)*cos(lamb)=Xe/2, (Rh+h)cos(phi)*sin(lamb)=Ye/2
  cos(lamb)/1 -> (Rh+h)cos(phi)*cos(lamb)=Xe/3
  sin(lamb)/1 -> (Rh+h)cos(phi)*sin(lamb)=Ye/3
  Ze/1 -> "Ze, m "/1
  Deg2R/1 -> cos(phi)/1, sin(phi)/1
  "Deg2R "/1 -> cos(lamb)/1, sin(lamb)/1
  Sum2/1 -> (Rh+h)cos(phi)*sin(lamb)=Ye/1, (Rh+h)cos(phi)*cos(lamb)=Xe/1
  (Rh+h)cos(phi)*cos(lamb)=Xe/1 -> "Xe, m "/1
  (Rh+h)cos(phi)*sin(lamb)=Ye/1 -> "Ye, m "/1

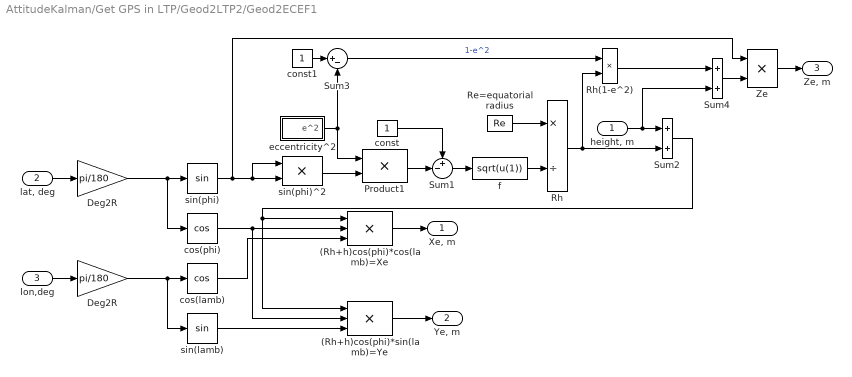
== system AttitudeKalman/Get GPS in LTP/Geod2LTP2/Geod2ECEF1 ==
  "height, m" : Inport
  "lat, deg" : Inport  Port=2
  lon,deg : Inport  Port=3
  (Rh+h)cos(phi)*cos(lamb)=Xe : Product  Inputs=3  SaturateOnIntegerOverflow=on  InputSameDT=on
  (Rh+h)cos(phi)*sin(lamb)=Ye : Product  Inputs=3  SaturateOnIntegerOverflow=on  InputSameDT=on
  Deg2R : Gain  Gain=pi/180  SaturateOnIntegerOverflow=on
  "Deg2R " : Gain  Gain=pi/180  SaturateOnIntegerOverflow=on
  Product1 : Product  SaturateOnIntegerOverflow=on  InputSameDT=on
  Re=equatorial radius : Constant  Value=Re
  Rh : Product  Inputs=*/  SaturateOnIntegerOverflow=on  InputSameDT=on
  Rh(1-e^2) : Product  SaturateOnIntegerOverflow=on  InputSameDT=on
  Sum1 : Sum  Inputs=+-|  SaturateOnIntegerOverflow=on  InputSameDT=on
  Sum2 : Sum  SaturateOnIntegerOverflow=on  InputSameDT=on
      settings: AttributesFormatString=Rh+h
  Sum3 : Sum  Inputs=|+-  SaturateOnIntegerOverflow=on  InputSameDT=on
  Sum4 : Sum  SaturateOnIntegerOverflow=on  InputSameDT=on
      settings: AttributesFormatString=(1-e^2)Rh+h
  Ze : Product  SaturateOnIntegerOverflow=on  InputSameDT=on
  const : Constant
  const1 : Constant
  cos(lamb) : Trigonometry  Operator=cos
  cos(phi) : Trigonometry  Operator=cos
  eccentricity^2 : Subsystem
  f : Fcn  Expr=sqrt(u(1))
  sin(lamb) : Trigonometry
  sin(phi) : Trigonometry
  sin(phi)^2 : Product  SaturateOnIntegerOverflow=on  InputSameDT=on
  "Xe, m " : Outport
  "Ye, m " : Outport  Port=2
  "Ze, m " : Outport  Port=3
  wires:
  (Rh+h)cos(phi)*sin(lamb)=Ye/1 -> "Ye, m "/1
  (Rh+h)cos(phi)*cos(lamb)=Xe/1 -> "Xe, m "/1
  Sum2/1 -> (Rh+h)cos(phi)*cos(lamb)=Xe/1, (Rh+h)cos(phi)*sin(lamb)=Ye/1
  "Deg2R "/1 -> sin(lamb)/1, cos(lamb)/1
  Deg2R/1 -> sin(phi)/1, cos(phi)/1
  Ze/1 -> "Ze, m "/1
  sin(lamb)/1 -> (Rh+h)cos(phi)*sin(lamb)=Ye/3
  cos(lamb)/1 -> (Rh+h)cos(phi)*cos(lamb)=Xe/3
  cos(phi)/1 -> (Rh+h)cos(phi)*sin(lamb)=Ye/2, (Rh+h)cos(phi)*cos(lamb)=Xe/2
  lon,deg/1 -> "Deg2R "/1
  Sum4/1 -> Ze/2
  Rh(1-e^2)/1 -> Sum4/1
  Sum3/1 -> Rh(1-e^2)/1  "1-e^2"
  const1/1 -> Sum3/1
  sin(phi)^2/1 -> Product1/2
  eccentricity^2/1(e^2) -> Sum3/2, Product1/1
  "height, m"/1 -> Sum2/1, Sum4/2
  const/1 -> Sum1/1
  Sum1/1 -> f/1
  Product1/1 -> Sum1/2
  Rh/1 -> Rh(1-e^2)/2, Sum2/2
  Re=equatorial radius/1 -> Rh/1
  f/1 -> Rh/2
  sin(phi)/1 -> Ze/1, sin(phi)^2/2, sin(phi)^2/1
  "lat, deg"/1 -> Deg2R/1

== system AttitudeKalman/Kalman Filter/GPS Update/Detect Change ==
  Data : Inport
  Abs1 : Abs
  Difference1 : simulink/Discrete/Difference  SystemSampleTime=-1  ICPrevInput=0.0  OutDataType=sfix(16)  OutScaling=2^-10  DoSatur=off
  Saturation1 : Saturate  UpperLimit=1  LowerLimit=0  SampleTime=SampleT
  change? : Outport
  wires:
  Difference1/1 -> Abs1/1
  Abs1/1 -> Saturation1/1
  Data/1 -> Difference1/1
  Saturation1/1 -> change?/1

== system AttitudeKalman/Kalman Filter/GPS Update/Detect Change1 ==
  Data : Inport
  Abs1 : Abs
  Difference1 : simulink/Discrete/Difference  SystemSampleTime=-1  ICPrevInput=0.0  OutDataType=sfix(16)  OutScaling=2^-10  DoSatur=off
  Saturation1 : Saturate  UpperLimit=1  LowerLimit=0  SampleTime=SampleT
  change? : Outport
  wires:
  Saturation1/1 -> change?/1
  Data/1 -> Difference1/1
  Abs1/1 -> Saturation1/1
  Difference1/1 -> Abs1/1

== system AttitudeKalman/Kalman Filter/GPS Update/Detect Change2 ==
  Data : Inport
  Abs1 : Abs
  Difference1 : simulink/Discrete/Difference  SystemSampleTime=-1  ICPrevInput=0.0  OutDataType=sfix(16)  OutScaling=2^-10  DoSatur=off
  Saturation1 : Saturate  UpperLimit=1  LowerLimit=0  SampleTime=SampleT
  change? : Outport
  wires:
  Difference1/1 -> Abs1/1
  Abs1/1 -> Saturation1/1
  Data/1 -> Difference1/1
  Saturation1/1 -> change?/1

== system AttitudeKalman/Kalman Filter/Measurement Update/Compute Gb ==
  SOG : Inport
  A : Inport  Port=2
  Vd : Inport  Port=3
  UpdateLat : Inport  Port=4
  COG : Inport  Port=5
  Constant1 : Constant  Value=ISA_g
  Divide : Product  Inputs=*//  OutScaling=2^-10
  Divide1 : Product  Multiplication=Matrix(*)  OutScaling=2^-10
  Embedded MATLAB Function : Stateflow chart
  Embedded MATLAB Function1 : Stateflow chart
  Integer Delay : simulink/Discrete/Integer Delay  vinit=0.0  samptime=-1  NumDelays=1
  Mux : Mux  Inputs=3
  Sum : Sum  Inputs=+-|
  Sum1 : Sum  Inputs=|+-
  Gb : Outport
  wires:
  Constant1/1 -> Divide/2
  Embedded MATLAB Function/1(Cnb) -> Divide1/1
  Divide/1 -> Divide1/2
  Divide1/1 -> Sum/2
  A/1 -> Sum/1
  COG/1 -> Embedded MATLAB Function/1(psi), Embedded MATLAB Function1/2(cog)
  Embedded MATLAB Function1/1(Vn) -> Mux/1
  Embedded MATLAB Function1/2(Ve) -> Mux/2
  Vd/1 -> Mux/3
  Mux/1 -> Sum1/1, Integer Delay/1
  Sum1/1 -> Divide/1
  Integer Delay/1 -> Sum1/2
  UpdateLat/1 -> Divide/3
  SOG/1 -> Embedded MATLAB Function1/1(sog)
  Sum/1 -> Gb/1

== system AttitudeKalman/Kalman Filter/Measurement Update/Compute qerr ==
  Euler : Inport
  qhat : Inport  Port=2
  Euler Angles to Quaternions : aerolibtransform2/Euler Angles to Quaternions  SystemSampleTime=-1
  Quaternion Inverse : aerolibutil/Quaternion Inverse  SystemSampleTime=-1
  Quaternion Multiplication : aerolibutil/Quaternion Multiplication  SystemSampleTime=-1
  qerr : Outport
  wires:
  qhat/1 -> Quaternion Inverse/1
  Quaternion Multiplication/1 -> qerr/1
  Euler Angles to Quaternions/1 -> Quaternion Multiplication/1
  Quaternion Inverse/1 -> Quaternion Multiplication/2
  Euler/1 -> Euler Angles to Quaternions/1

== system AttitudeKalman/Kalman Filter/Measurement Update/Get Phi Theta ==
  Gb : Inport
  Demux : Demux  Outputs=3
  Gain : Gain  Gain=-1
  Saturation : Saturate  UpperLimit=1  LowerLimit=-1
  Saturation1 : Saturate  UpperLimit=1  LowerLimit=-1
  Terminator : Terminator
  Trigonometric Function : Trigonometry  Operator=asin
  Trigonometric Function1 : Trigonometry  Operator=asin
  Phi : Outport
  Theta : Outport  Port=2
  wires:
  Demux/2 -> Saturation/1
  Trigonometric Function/1 -> Gain/1
  Saturation/1 -> Trigonometric Function/1
  Saturation1/1 -> Trigonometric Function1/1
  Demux/1 -> Saturation1/1
  Demux/3 -> Terminator/1
  Trigonometric Function1/1 -> Theta/1
  Gb/1 -> Demux/1
  Gain/1 -> Phi/1

== system AttitudeKalman/Kalman Filter/Measurement Update/Update  L and P ==
  P : Inport
  Constant1 : Constant  Value=H
  Divide1 : Product  Multiplication=Matrix(*)  OutScaling=2^-10
  Divide2 : Product  Multiplication=Matrix(*)  OutScaling=2^-10
  Identity Matrix : dspmtrx3/Identity Matrix  Inherit=off  N=6  Ts=SampleT  dataType=double  isSigned=on  wordLen=16  udDataType=sfix(16)  fracBitsMode=Best precision  numFracBits=15
  Kalman Gain : Subsystem
  Sum : Sum  Inputs=|-+
  L : Outport
  P(+) : Outport  Port=2
  wires:
  P/1 -> Kalman Gain/1(P), Divide1/2
  Kalman Gain/1(L) -> L/1, Divide2/1
  Constant1/1 -> Divide2/2
  Divide2/1 -> Sum/1
  Identity Matrix/1 -> Sum/2
  Sum/1 -> Divide1/1
  Divide1/1 -> P(+)/1

== system AttitudeKalman/Kalman Filter/Time Update/Subsystem ==
  Constant : Constant  Value=Rwpsd./SampleT
  Constant1 : Constant  Value=Gw
  Constant2 : Constant  Value=Gw
  Divide : Product  Inputs=3  Multiplication=Matrix(*)  OutScaling=2^-10
  Transpose : dspmtrx3/Transpose  SystemSampleTime=-1  Hermitian=off  overflowFlag=off
  Cd : Outport
  wires:
  Constant2/1 -> Transpose/1
  Constant1/1 -> Divide/1
  Constant/1 -> Divide/2
  Transpose/1 -> Divide/3
  Divide/1 -> Cd/1

== system AttitudeKalman/Plant Model/Plant/6-DOF EOM ==
  "[F,M]" : Inport
  Vb Corr : Inport  Orientation=left  Port=2
  Angular Rates : Integrator  InitialCondition=PQR_0'
  Demux1 : Demux  Outputs=2
  Display1 : Display
  Euler Angles : Integrator  InitialCondition=Euler_0
  Get Euler Dot : Subsystem
      mask Display:
      | port_label('input', 1, 'p, q, r')
      | port_label('input', 2, 'Euler')
      | port_label('output', 1, 'Euler_dot')
  Mux : Mux  Orientation=left  Inputs=[3;3]
  NED2NEU : Gain  Gain=[1 0 0;0 1 0;0 0 -1]  Multiplication=Matrix(K*u)  SaturateOnIntegerOverflow=on
  Position : Integrator  InitialCondition=Pos_0'
  RB2L * Vb : Product  Multiplication=Matrix(*)  SaturateOnIntegerOverflow=on  InputSameDT=on
  RB2LTP : Subsystem
  Velocities Body : Integrator  InitialCondition=Vb_0'
  "[V1,2,3,W1,2,3]" : Subsystem
  X,Y,Z (LTP) NEU : Outport
  "Vx, Vy, Vz [NED]" : Outport  Port=2
  Euler : Outport  Port=3
  "p, q, r" : Outport  Orientation=left  Port=4
  Euler_dot : Outport  Port=5
  A_b : Outport  Port=6
  A_bMeas : Outport  Port=7
  wires:
  Euler Angles/1 -> RB2LTP/1(Euler), Euler/1, Get Euler Dot/2(Euler), "[V1,2,3,W1,2,3]"/2(Euler)
  Demux1/1 -> Velocities Body/1, A_b/1, Display1/1
  "[V1,2,3,W1,2,3]"/2(V*dot) -> Demux1/1
  Demux1/2 -> Angular Rates/1
  "[F,M]"/1 -> "[V1,2,3,W1,2,3]"/1("[F ; M]")
  RB2LTP/1(Rot) -> RB2L * Vb/1
  Velocities Body/1 -> RB2L * Vb/2
  Position/1 -> X,Y,Z (LTP) NEU/1
  Angular Rates/1 -> Get Euler Dot/1(p,q,r), Mux/2, "p, q, r"/1
  RB2L * Vb/1 -> NED2NEU/1, "Vx, Vy, Vz [NED]"/1  "NED"
  NED2NEU/1 -> Position/1
  Get Euler Dot/1(Euler_dot) -> Euler Angles/1, Euler_dot/1
  Vb Corr/1 -> Mux/1
  Mux/1 -> "[V1,2,3,W1,2,3]"/3(V*)
  "[V1,2,3,W1,2,3]"/1("Acc_meas ") -> A_bMeas/1

== system AttitudeKalman/Plant Model/Plant/Engine Model ==
  dt : Inport
  Vmag : Inport  Port=2
  Constant4 : Constant  Value=0  SampleTime=SampleT
  Get To1 : Subsystem
  Mux : Mux  Inputs=2
  Mux1 : Mux  Inputs=3
  Thrust Available (lbs) : Fcn  Expr=u(1) - 0.047*sqrt(u(1))*u(2)
  kg2N : Gain  Gain=ISA_g  SaturateOnIntegerOverflow=on
  lbs2kg : Gain  Gain=0.45359237  SaturateOnIntegerOverflow=on
  RPM : Outport
  Thrust : Outport  Port=2
  wires:
  kg2N/1 -> Mux1/1
  Constant4/1 -> Mux1/3, Mux1/2
  lbs2kg/1 -> kg2N/1
  Mux1/1 -> Thrust/1
  Vmag/1 -> Mux/2
  Thrust Available (lbs)/1 -> lbs2kg/1
  Mux/1 -> Thrust Available (lbs)/1
  Get To1/2(To) -> Mux/1
  dt/1 -> Get To1/1(dt)
  Get To1/1(RPM) -> RPM/1

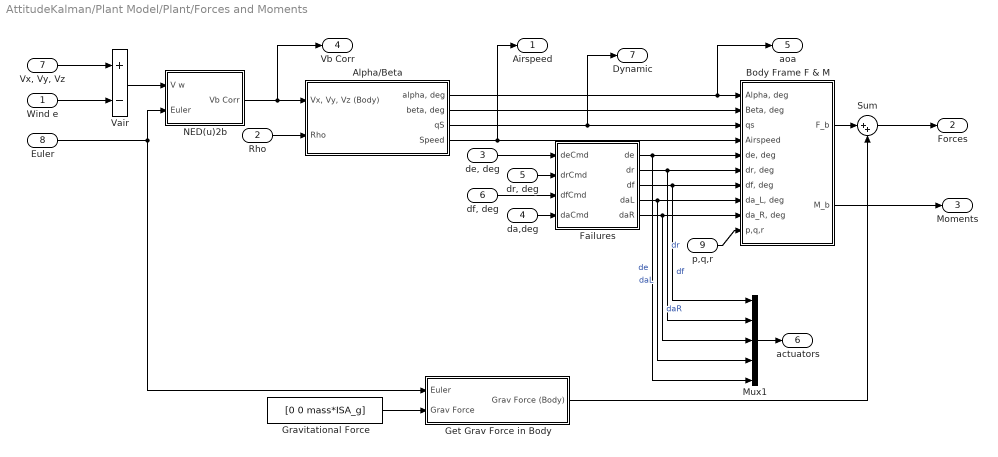
== system AttitudeKalman/Plant Model/Plant/Forces and Moments ==
  Wind e : Inport
  Rho : Inport  Port=2
  "de, deg" : Inport  Port=3
  da,deg : Inport  Port=4
  "dr, deg" : Inport  Port=5
  "df, deg" : Inport  Port=6
  "Vx, Vy, Vz " : Inport  Port=7
  Euler : Inport  Port=8  PortDimensions=3
  p,q,r : Inport  Port=9
  Alpha/Beta : Subsystem
  Body Frame F & M : Subsystem
  Failures : Subsystem
  Get Grav Force in Body : Subsystem
  Gravitational Force : Constant  Value=[0 0 mass*ISA_g]  VectorParams1D=off
  Mux1 : Mux  Inputs=5
  NED(u)2b : Subsystem
  Sum : Sum  Inputs=|++  SaturateOnIntegerOverflow=on
  Vair : Sum  Inputs=+-  SaturateOnIntegerOverflow=on  InputSameDT=on
  Airspeed : Outport
  Forces : Outport  Port=2
  Moments : Outport  Port=3
  Vb Corr : Outport  Port=4
  aoa : Outport  Port=5
  actuators : Outport  Port=6
  Dynamic : Outport  Port=7
  wires:
  "Vx, Vy, Vz "/1 -> Vair/1
  Vair/1 -> NED(u)2b/1(V w)
  Euler/1 -> NED(u)2b/2(Euler), Get Grav Force in Body/1(Euler)
  Rho/1 -> Alpha/Beta/2(Rho)
  NED(u)2b/1(Vb Corr) -> Alpha/Beta/1("Vx, Vy, Vz (Body)"), Vb Corr/1
  Body Frame F & M/2(M_b) -> Moments/1
  Gravitational Force/1 -> Get Grav Force in Body/2(Grav Force)
  Body Frame F & M/1(F_b) -> Sum/1
  Sum/1 -> Forces/1
  Get Grav Force in Body/1(Grav Force (Body)) -> Sum/2
  Alpha/Beta/3(qS) -> Body Frame F & M/3(qs), Dynamic/1
  Alpha/Beta/4(Speed) -> Body Frame F & M/4(Airspeed), Airspeed/1
  p,q,r/1 -> Body Frame F & M/10(p,q,r)
  Alpha/Beta/2("beta, deg") -> Body Frame F & M/2("Beta, deg")
  Alpha/Beta/1("alpha, deg") -> Body Frame F & M/1("Alpha, deg"), aoa/1
  Wind e/1 -> Vair/2
  Mux1/1 -> actuators/1
  Failures/1(de) -> Body Frame F & M/5("de, deg"), Mux1/5  "de"
  Failures/2(dr) -> Body Frame F & M/6("dr, deg"), Mux1/2  "dr"
  Failures/3(df) -> Body Frame F & M/7("df, deg"), Mux1/1  "df"
  Failures/4(daL) -> Body Frame F & M/8("da_L, deg"), Mux1/4  "daL"
  Failures/5(daR) -> Body Frame F & M/9("da_R, deg"), Mux1/3  "daR"
  "de, deg"/1 -> Failures/1(deCmd)
  "dr, deg"/1 -> Failures/2(drCmd)
  "df, deg"/1 -> Failures/3(dfCmd)
  da,deg/1 -> Failures/4(daCmd)

== system AttitudeKalman/Plant Model/Plant/Get GPS ==
  XYZ (NEU) : Inport
  Angle Conversion : aerolibconvert2/Angle Conversion  SystemSampleTime=-1  IU=deg  OU=rad
  Demux : Demux  Outputs=6
  Demux2 : Demux  Outputs=2
  Flat Earth to LLA : aerolibtransform2/Flat Earth to LLA  SystemSampleTime=-1  units=Metric (MKS)  ptype=Earth (WGS84)  F=1/298.257223563  R=6378137  LL0=[37.0004768371582, -122.061897277832]  psi=0
  MATLAB Fcn : MATLABFcn  MATLABFcn=u(1)*clock  OutputSignalType=real
  NEU2NED : Gain  Gain=[1 0 0;0 1 0;0 0 -1]  Multiplication=Matrix(K*u)  SaturateOnIntegerOverflow=on
  Rounding Function : Rounding
  Zero level trust : Constant  Value=0
  Zero level trust1 : Constant
  Zero level trust2 : Constant  Value=0
  GPS Month : Outport
  GPS Day : Outport  Port=2
  GPS Year : Outport  Port=3
  GPS Hr : Outport  Port=4
  GPS Min : Outport  Port=5
  GPS Sec : Outport  Port=6
  GPS Frac Sec : Outport  Port=7
  GPS Lat (rad) : Outport  Port=8
  GPS Long (rad) : Outport  Port=9
  GPS H (m) : Outport  Port=10
  wires:
  NEU2NED/1 -> Flat Earth to LLA/1
  Zero level trust/1 -> Flat Earth to LLA/2
  XYZ (NEU)/1 -> NEU2NED/1
  Flat Earth to LLA/1 -> Angle Conversion/1
  Flat Earth to LLA/2 -> GPS H (m)/1
  Zero level trust1/1 -> MATLAB Fcn/1
  MATLAB Fcn/1 -> Demux/1
  Demux/2 -> GPS Month/1
  Demux/3 -> GPS Day/1
  Demux/1 -> GPS Year/1
  Demux/4 -> GPS Hr/1
  Demux/5 -> GPS Min/1
  Demux/6 -> Rounding Function/1
  Rounding Function/1 -> GPS Sec/1
  Zero level trust2/1 -> GPS Frac Sec/1
  Angle Conversion/1 -> Demux2/1
  Demux2/1 -> GPS Lat (rad)/1
  Demux2/2 -> GPS Long (rad)/1

== system AttitudeKalman/Plant Model/Plant/ISA Atmosphere & Winds ==
  "X, Y, Z" : Inport  SampleTime=APtsamp
  Correct Wind : Constant  Value=[0;0;0]  SampleTime=APtsamp
  Get Z : Selector  IndexOptions=Index vector (dialog)  Indices=[3]  OutputSizes=[(-2)]  InputPortWidth=3
  ISA Atmosphere Model1 : aerolibatmos2/ISA Atmosphere Model  SystemSampleTime=-1  custom=off  g=9.80665  gamma=1.4  R=287.0531  L=0.0065  h_trop=11000  h_strat=20000  rho0=1.225  P0=101325  T0=288.15
  Temperature Conversion : aerolibconvert2/Temperature Conversion  SystemSampleTime=-1  IU=K  OU=C
  Terminator1 : Terminator
  Rho : Outport
  Wind : Outport  Port=2
  OAT (C) : Outport  Port=3
  Static (Pa) : Outport  Port=4
  wires:
  "X, Y, Z"/1 -> Get Z/1
  Get Z/1 -> ISA Atmosphere Model1/1
  ISA Atmosphere Model1/4 -> Rho/1
  ISA Atmosphere Model1/1 -> Temperature Conversion/1
  ISA Atmosphere Model1/2 -> Terminator1/1
  ISA Atmosphere Model1/3 -> Static (Pa)/1
  Correct Wind/1 -> Wind/1
  Temperature Conversion/1 -> OAT (C)/1

== system AttitudeKalman/Get GPS in LTP/Geod2LTP2/ECEF2LTP (UEN)/From Body to Universal1 ==
  long : Inport
  lat : Inport  Port=2
  Mux : Mux  Inputs=2
  Reshape 9x1->3x1 : S-Function  FunctionName=sreshape  Parameters=OutputDimensionality, OutputDimensions  mask(Reshape){OutputDimensionality=Customize, OutputDimensions=[3,3]}
      mask prompts: OutputDimensionality "Output dimensionality:"; OutputDimensions "Output dimensions:"
      mask help:
      | Change the dimensions of a vector or matrix input signal. Output
      |  - a one-dimensional array (vector),
      |  - a column vector (Mx1 matrix),
      |  - a row vector (1xN matrix), or
      |  - a matrix or vector with specified dimensions, e.g., [M, N] or [W].
      mask init:
      | s = reshapemask(gcb,'init');
      mask StyleString: popup(1-D array|Column vector|Row vector|Customize),edit
      mask CallbackString: reshapemask(gcb,'cbDimensionality')|
      mask Display: disp('Reshape')
  Rotation Matrix from Long//Lat : Subsystem
      mask Type: Vector Transformation
      mask Description: Vector Transformation
      mask Display: disp('axis')
  DCM : Outport
  wires:
  lat/1 -> Mux/2
  long/1 -> Mux/1
  Mux/1 -> Rotation Matrix from Long//Lat/1(long lat)
  Rotation Matrix from Long//Lat/1(DCM) -> Reshape 9x1->3x1/1
  Reshape 9x1->3x1/1 -> DCM/1

== system AttitudeKalman/Get GPS in LTP/Geod2LTP2/Geod2ECEF/eccentricity^2 ==
  " " : Product  SaturateOnIntegerOverflow=on  InputSameDT=on
  Re=equatorial radius1 : Constant  Value=Re
  Rp=polar radius : Constant  Value=Rp
  Sum5 : Sum  Inputs=|+-  SaturateOnIntegerOverflow=on  InputSameDT=on
  const2 : Constant
  e^1 : Product  Inputs=*/  SaturateOnIntegerOverflow=on  InputSameDT=on
  e^2 : Outport
  wires:
  Re=equatorial radius1/1 -> e^1/2
  Rp=polar radius/1 -> e^1/1
  const2/1 -> Sum5/1
  e^1/1 -> " "/2, " "/1
  " "/1 -> Sum5/2
  Sum5/1 -> e^2/1

== system AttitudeKalman/Get GPS in LTP/Geod2LTP2/Geod2ECEF1/eccentricity^2 ==
  " " : Product  SaturateOnIntegerOverflow=on  InputSameDT=on
  Re=equatorial radius1 : Constant  Value=Re
  Rp=polar radius : Constant  Value=Rp
  Sum5 : Sum  Inputs=|+-  SaturateOnIntegerOverflow=on  InputSameDT=on
  const2 : Constant
  e^1 : Product  Inputs=*/  SaturateOnIntegerOverflow=on  InputSameDT=on
  e^2 : Outport
  wires:
  Sum5/1 -> e^2/1
  " "/1 -> Sum5/2
  e^1/1 -> " "/1, " "/2
  const2/1 -> Sum5/1
  Rp=polar radius/1 -> e^1/1
  Re=equatorial radius1/1 -> e^1/2

== system AttitudeKalman/Kalman Filter/Measurement Update/Update  L and P/Kalman Gain ==
  P : Inport
  Cholesky Inverse : dspinverses/Cholesky Inverse  SystemSampleTime=-1  errmode=Warning
  Constant : Constant  Value=transpose(H)
  Constant1 : Constant  Value=H
  Constant2 : Constant  Value=Rv
  Divide : Product  Multiplication=Matrix(*)  OutScaling=2^-10
  Divide1 : Product  Multiplication=Matrix(*)  OutScaling=2^-10
  Divide2 : Product  Multiplication=Matrix(*)  OutScaling=2^-10
  Sum : Sum  Inputs=|++
  L : Outport
  wires:
  Divide/1 -> Sum/1
  Constant2/1 -> Sum/2
  Sum/1 -> Cholesky Inverse/1
  Divide2/1 -> Divide/2, Divide1/1
  P/1 -> Divide2/1
  Constant/1 -> Divide2/2
  Constant1/1 -> Divide/1
  Cholesky Inverse/1 -> Divide1/2
  Divide1/1 -> L/1
